simulink model "Test2"  (R2017b)
settings: Solver=ode23tb  StartTime=0.0  StopTime=6  MaxStep=1e-4  RelTol=1e-3
undefined symbols (not defined in the file): DiscIntNeverNeededParam
libraries: powerlib x5, simulink x1
settings Model: Creator=80573  LastModifiedBy=80573

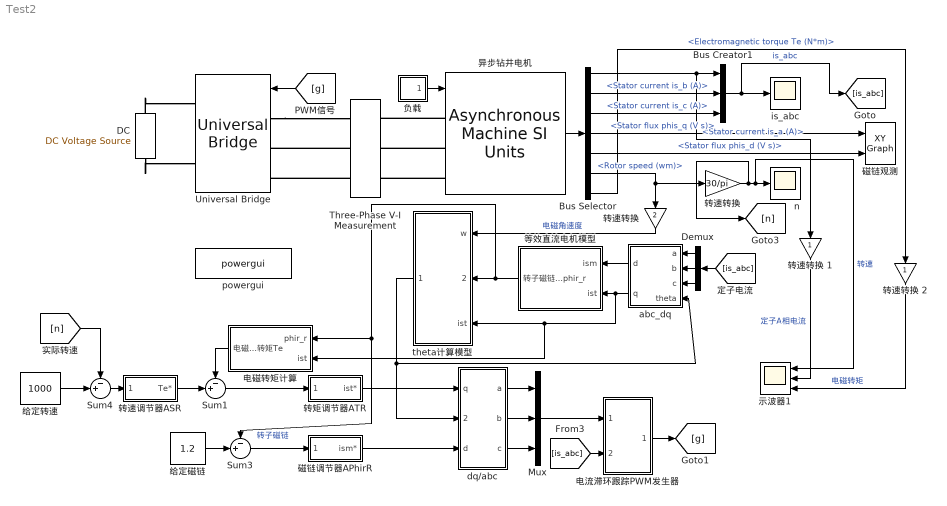
== system Test2 ==
  Bus Creator1 : BusCreator  Inputs=3
  Bus Selector : BusSelector  OutputSignals=Stator measurements.Stator current is_a (A),Stator measurements.Stator current is_b (A),Stator measurements.Stator current is_c (A),Stator measurements.Stator flux phis_q (V s),Stator measurements.Stator flux phis_d (V s),Mechanical.Rotor speed (wm),Mechanical.Electromagnetic torque Te (N*m)
  DC : powerlib/Electrical Sources/DC Voltage Source  Amplitude=510  Measurements=None
  Demux : Demux  Outputs=3
  Mux : Mux  Inputs=3
  Sum1 : Sum  Inputs=-+|
  Sum3 : Sum  Inputs=-+|
  Sum4 : Sum  Inputs=-+|
  Three-Phase V-I Measurement : powerlib/Measurements/Three-Phase V-I Measurement  VoltageMeasurement=phase-to-phase  SetLabelV=on  LabelV=Vabc  Vpu=off  VpuLL=off  CurrentMeasurement=yes  SetLabelI=on  LabelI=Iabc  Ipu=off  Pbase=100e6  Vbase=500e3  OutputType=Complex  PhasorSimulation=off  PSBequivalent=0
  Universal Bridge : powerlib/Power Electronics/Universal Bridge  Arms=3  SnubberResistance=1e5  SnubberCapacitance=inf  Device=IGBT / Diodes  Ron=1e-3  Lon=0  ForwardVoltages="[  0  0  ]"  ForwardVoltage=0  GTOparameters=[ 10e-6 , 20e-6 ]  IGBTparameters=[ 1e-6 , 2e-6 ]  Measurements=None  Measurements_2=None  converterType=Rectifier
  abc_dq : Subsystem
  dq/abc : Subsystem
  is_abc : Scope
  n : Scope
  powergui : powerlib/powergui  SimulationMode=Discrete  SampleTime=0.00001  frequency=50  Iterations=50  frequencyindice=0  Pbase=100e6  ErrMax=1e-4  UnitsV=kV  UnitsW=MW  buscounter=0  FunctionMessages=off  echomessages=off  EnableUseOfTLC=off  CurrentSourceSwitches=off  DisableSnubberDevices=off  DisableRonSwitches=off  DisableVfSwitches=off  DisplayEquations=off  SolverType=Tustin/Backward Euler (TBE)  Interpol=off  ExternalGateDelay=off  methode=off  Ts=100  x0status=zero  SPID=on  SwTol=0  HookPort=off  RestoreLinks=warning  ResistiveCurrentMeasurement=off  Frange=[0:2:500]  Ylog=off  Xlog=on  ShowGrid=off  save=off  variable=ZData  structure=0  ZoomFFT=on  StartTime=0.0  cycles=1  DisplayStyle=1  fundamental=60  FreqAxis=off  MaxFrequency=1000  frequencyindicesteady=1  RmsSteady=1  display=off
  theta计算模型 : Subsystem
  异步钻井电机 : powerlib/Machines/Asynchronous Machine SI Units  RotorType=Squirrel-cage  PresetModel=No  MechanicalLoad=Torque Tm  ShowDetailedParameters=on  ReferenceFrame=Stationary  Units=SI  MeasurementBus=off  NominalParameters=[149200 380 50]  Stator=[0.01485 0.0003027]  Rotor=[0.05295 0.0003027]  Cage1=[0.4155 0.002066]  Cage2=[0.4168 0.0003495]  Lm=0.01046  Mechanical=[3.1 0.08 2]  PolePairs=2  InitialConditions=[1 0 0 0 0 0 0 0]  SimulateSaturation=off  Saturation=[14.03593122, 27.81365428, 53.79336849, 72.68890987, 97.98006896, 148.6815601, 215.7428561, 302.9841135, 428.7778367 ; 230, 322, 414, 460, 506, 552, 598, 644, 690]  LoadFlowParameters=1492000  TsPowergui=0  TsBlock=-1  IterativeModel=Trapezoidal non iterative  IterativeDiscreteModel=Trapezoidal non iterative  Pmec=1.492e+006
  电流滞环跟踪PWM发生器 : Subsystem
  电磁转矩计算 : Subsystem
  磁链观测 : simulink/Sinks/XY Graph  xmin=-1  xmax=1  ymin=-1  ymax=1  st=-1
  磁链调节器APhirR : Subsystem
  示波器1 : Scope  NumInputPorts=3
  等效直流电机模型 : Subsystem
  给定磁链 : Constant  Value=1.2
  给定转速 : Constant  Value=1000
  负载 : Subsystem
  转矩调节器ATR : Subsystem
  转速调节器ASR : Subsystem
  转速转换 : Gain  Gain=30/pi
  "转速转换 " : Gain  Gain=2
  转速转换 1 : Gain
  转速转换 2 : Gain
  wires:
  Bus Selector/7 -> 转速转换 2/1  "<Electromagnetic torque Te (N*m)>"
  Demux/3 -> abc_dq/3(c)
  Sum1/1 -> 转矩调节器ATR/1(" ")
  转矩调节器ATR/1(ist*) -> dq/abc/1(q)
  [n] -> Sum4/1
  "转速转换 "/1 -> theta计算模型/1(w)  "电磁角速度"
  电流滞环跟踪PWM发生器/1(pulse) -> [g]
  Bus Selector/5 -> 磁链观测/2  "<Stator flux phis_d (V s)>"
  Sum4/1 -> 转速调节器ASR/1("  ")
  dq/abc/1(a) -> Mux/1
  转速转换/1 -> [n], 示波器1/1, n/1  "转速"
  dq/abc/2(b) -> Mux/2
  转速转换 2/1 -> 示波器1/3  "电磁转矩"
  异步钻井电机/1 -> Bus Selector/1
  theta计算模型/1(theta) -> dq/abc/2(theta), abc_dq/4(theta)
  Bus Selector/6 -> 转速转换/1, "转速转换 "/1  "<Rotor speed (wm)>"
  转速调节器ASR/1(Te*) -> Sum1/2
  Bus Selector/2 -> Bus Creator1/2  "<Stator current is_b (A)>"
  电磁转矩计算/1(电磁转矩Te) -> Sum1/1
  abc_dq/1(d) -> 等效直流电机模型/1(ism)
  负载/1(TL) -> 异步钻井电机/1
  Mux/1 -> 电流滞环跟踪PWM发生器/1(Iabc*)
  Demux/2 -> abc_dq/2(b)
  [is_abc] -> Demux/1
  [is_abc] -> 电流滞环跟踪PWM发生器/2(Iabc)
  dq/abc/3(c) -> Mux/3
  转速转换 1/1 -> 示波器1/2  "定子A相电流"
  Bus Selector/1 -> 转速转换 1/1, Bus Creator1/1  "<Stator current is_a (A)>"
  abc_dq/2(q) -> 等效直流电机模型/2(ist), theta计算模型/3(ist), 电磁转矩计算/2(ist)
  Bus Selector/3 -> Bus Creator1/3  "<Stator current is_c (A)>"
  Demux/1 -> abc_dq/1(a)
  给定磁链/1 -> Sum3/2
  Sum3/1 -> 磁链调节器APhirR/1(" ")
  Bus Selector/4 -> 磁链观测/1  "<Stator flux phis_q (V s)>"
  Bus Creator1/1 -> is_abc/1, [is_abc]  "is_abc"
  磁链调节器APhirR/1(ism*) -> dq/abc/3(d)
  [g] -> Universal Bridge/1
  等效直流电机模型/1(转子磁链phir_r) -> theta计算模型/2(phir_r), Sum3/1, 电磁转矩计算/1(phir_r)  "转子磁链"
  给定转速/1 -> Sum4/2
  connections:
  DC/LConn1 -- Universal Bridge/RConn2
  Three-Phase V-I Measurement/LConn3 -- Universal Bridge/LConn3
  异步钻井电机/LConn2 -- Three-Phase V-I Measurement/RConn2
  异步钻井电机/LConn3 -- Three-Phase V-I Measurement/RConn3
  Universal Bridge/LConn1 -- Three-Phase V-I Measurement/LConn1
  DC/RConn1 -- Universal Bridge/RConn1
  Three-Phase V-I Measurement/LConn2 -- Universal Bridge/LConn2
  异步钻井电机/LConn1 -- Three-Phase V-I Measurement/RConn1

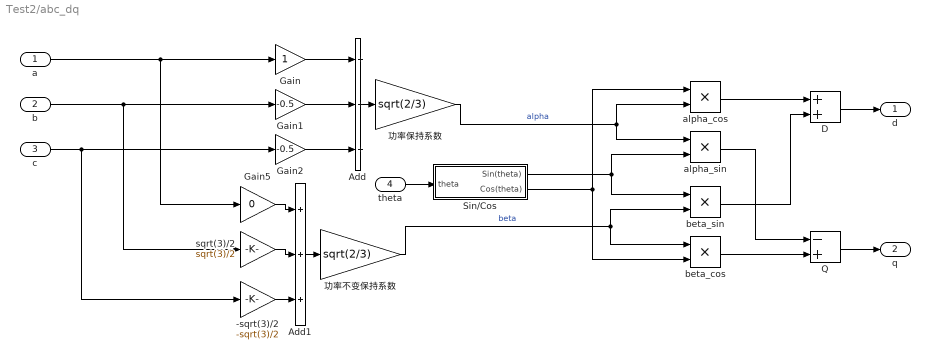
== system Test2/abc_dq ==
  a : Inport
  b : Inport  Port=2
  c : Inport  Port=3
  theta : Inport  Port=4
  -sqrt(3)/2 : Gain  Gain=-sqrt(3)/2
  Add : Sum  Inputs=3
  Add1 : Sum  Inputs=3
  D : Sum
  Gain : Gain
  Gain1 : Gain  Gain=-0.5
  Gain2 : Gain  Gain=-0.5
  Gain5 : Gain  Gain=0
  Q : Sum  Inputs=-+
  Sin/Cos : Subsystem
  alpha_cos : Product
  alpha_sin : Product
  beta_cos : Product
  beta_sin : Product
  sqrt(3)/2 : Gain  Gain=sqrt(3)/2
  功率不变保持系数 : Gain  Gain=sqrt(2/3)
  功率保持系数 : Gain  Gain=sqrt(2/3)
  d : Outport
  q : Outport  Port=2
  wires:
  功率不变保持系数/1 -> beta_cos/1, beta_sin/2  "beta"
  D/1 -> d/1
  Sin/Cos/2(Cos(theta)) -> beta_cos/2, alpha_cos/1
  alpha_sin/1 -> Q/1
  Q/1 -> q/1
  beta_sin/1 -> D/2
  beta_cos/1 -> Q/2
  Sin/Cos/1(Sin(theta)) -> beta_sin/1, alpha_sin/2
  功率保持系数/1 -> alpha_cos/2, alpha_sin/1  "alpha"
  Add1/1 -> 功率不变保持系数/1
  c/1 -> Gain2/1, -sqrt(3)/2/1
  a/1 -> Gain5/1, Gain/1
  Gain2/1 -> Add/3
  sqrt(3)/2/1 -> Add1/2
  theta/1 -> Sin/Cos/1(theta)
  b/1 -> sqrt(3)/2/1, Gain1/1
  -sqrt(3)/2/1 -> Add1/3
  Gain1/1 -> Add/2
  Gain5/1 -> Add1/1
  alpha_cos/1 -> D/1
  Add/1 -> 功率保持系数/1
  Gain/1 -> Add/1

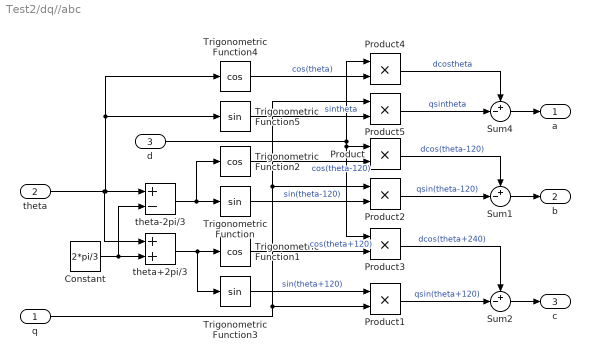
== system Test2/dq//abc ==
  q : Inport
  theta : Inport  Port=2
  d : Inport  Port=3
  Constant : Constant  Value=2*pi/3
  Product{,1..5} (6 alike) : Product
  Sum1 : Sum  Inputs=+-|
  Sum2 : Sum  Inputs=+-|
  Sum4 : Sum  Inputs=+-|
  Trigonometric Function : Trigonometry
  Trigonometric Function1 : Trigonometry  Operator=cos
  Trigonometric Function2 : Trigonometry  Operator=cos
  Trigonometric Function3 : Trigonometry
  Trigonometric Function4 : Trigonometry  Operator=cos
  Trigonometric Function5 : Trigonometry
  theta+2pi/3 : Sum
  theta-2pi/3 : Sum  Inputs=+-
  a : Outport
  b : Outport  Port=2
  c : Outport  Port=3
  wires:
  Trigonometric Function5/1 -> Product5/2  "sintheta"
  Product/1 -> Sum1/1  "dcos(theta-120)"
  Trigonometric Function1/1 -> Product3/2  "cos(theta+120)"
  Product3/1 -> Sum2/1  "dcos(theta+240)"
  d/1 -> Product/1, Product3/1, Product4/1
  Constant/1 -> theta+2pi/3/2, theta-2pi/3/2
  theta/1 -> Trigonometric Function4/1, Trigonometric Function5/1, theta-2pi/3/1, theta+2pi/3/1
  theta+2pi/3/1 -> Trigonometric Function3/1, Trigonometric Function1/1
  q/1 -> Product5/1, Product2/1, Product1/2
  Trigonometric Function/1 -> Product2/2  "sin(theta-120)"
  Product4/1 -> Sum4/1  "dcostheta"
  Product5/1 -> Sum4/2  "qsintheta"
  theta-2pi/3/1 -> Trigonometric Function2/1, Trigonometric Function/1
  Product1/1 -> Sum2/2  "qsin(theta+120)"
  Trigonometric Function2/1 -> Product/2  "cos(theta-120)"
  Sum4/1 -> a/1
  Sum1/1 -> b/1
  Trigonometric Function4/1 -> Product4/2  "cos(theta)"
  Trigonometric Function3/1 -> Product1/1  "sin(theta+120)"
  Product2/1 -> Sum1/2  "qsin(theta-120)"
  Sum2/1 -> c/1

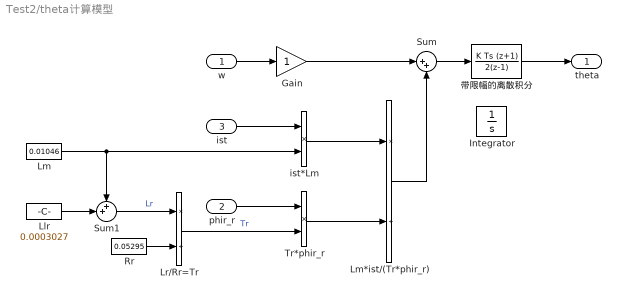
== system Test2/theta计算模型 ==
  w : Inport
  phir_r : Inport  Port=2
  ist : Inport  Port=3
  Gain : Gain
  Integrator : Integrator
  Llr : Constant  Value=0.0003027
  Lm : Constant  Value=0.01046
  Lm*ist/(Tr*phir_r) : Product  Inputs=*/
  Lr/Rr=Tr : Product  Inputs=*/
  Rr : Constant  Value=0.05295
  Sum : Sum  Inputs=|++
  Sum1 : Sum  Inputs=++|
  Tr*phir_r : Product
  ist*Lm : Product
  带限幅的离散积分 : DiscreteIntegrator  IntegratorMethod=Integration: Trapezoidal  SampleTime=2e-5  LimitOutput=on  UpperSaturationLimit=3000  LowerSaturationLimit=-3000  ICPrevOutput=DiscIntNeverNeededParam  ICPrevScaledInput=DiscIntNeverNeededParam
  theta : Outport
  wires:
  ist*Lm/1 -> Lm*ist/(Tr*phir_r)/1
  Lm*ist/(Tr*phir_r)/1 -> Sum/2
  Sum/1 -> 带限幅的离散积分/1
  w/1 -> Gain/1
  带限幅的离散积分/1 -> theta/1
  Lr/Rr=Tr/1 -> Tr*phir_r/2  "Tr"
  Lm/1 -> Sum1/1, ist*Lm/2
  Tr*phir_r/1 -> Lm*ist/(Tr*phir_r)/2
  ist/1 -> ist*Lm/1
  phir_r/1 -> Tr*phir_r/1
  Rr/1 -> Lr/Rr=Tr/2
  Gain/1 -> Sum/1
  Sum1/1 -> Lr/Rr=Tr/1  "Lr"
  Llr/1 -> Sum1/2

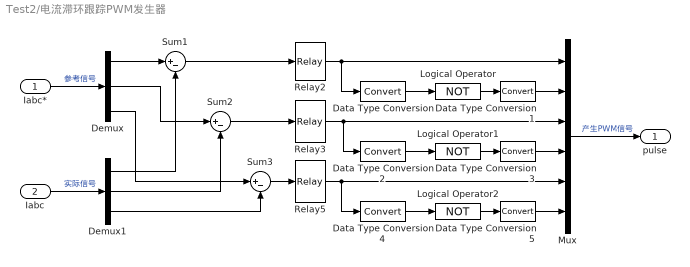
== system Test2/电流滞环跟踪PWM发生器 ==
  Iabc* : Inport
  Iabc : Inport  Port=2
  Data Type Conversion{,1..5} (6 alike) : DataTypeConversion
  Demux : Demux  Outputs=3
  Demux1 : Demux  Outputs=3
  Logical Operator : Logic  Operator=NOT  Inputs=1  AllPortsSameDT=off
  Logical Operator1 : Logic  Operator=NOT  Inputs=1  AllPortsSameDT=off
  Logical Operator2 : Logic  Operator=NOT  Inputs=1  AllPortsSameDT=off
  Mux : Mux  Inputs=6
  Relay2 : Relay  OnSwitchValue=0.2  OffSwitchValue=-0.2  ZeroCross=off
  Relay3 : Relay  OnSwitchValue=0.2  OffSwitchValue=-0.2  ZeroCross=off
  Relay5 : Relay  OnSwitchValue=0.2  OffSwitchValue=-0.2  ZeroCross=off
  Sum1 : Sum  Inputs=|+-
  Sum2 : Sum  Inputs=|+-
  Sum3 : Sum  Inputs=|+-
  pulse : Outport
  wires:
  Relay2/1 -> Data Type Conversion/1, Mux/1
  Data Type Conversion/1 -> Logical Operator/1
  Logical Operator/1 -> Data Type Conversion1/1
  Data Type Conversion1/1 -> Mux/2
  Mux/1 -> pulse/1  "产生PWM信号"
  Sum1/1 -> Relay2/1
  Demux/1 -> Sum1/1
  Demux1/3 -> Sum3/2
  Iabc/1 -> Demux1/1  "实际信号"
  Iabc*/1 -> Demux/1  "参考信号"
  Sum2/1 -> Relay3/1
  Logical Operator1/1 -> Data Type Conversion3/1
  Data Type Conversion3/1 -> Mux/4
  Data Type Conversion2/1 -> Logical Operator1/1
  Relay3/1 -> Data Type Conversion2/1, Mux/3
  Logical Operator2/1 -> Data Type Conversion5/1
  Data Type Conversion5/1 -> Mux/6
  Data Type Conversion4/1 -> Logical Operator2/1
  Relay5/1 -> Data Type Conversion4/1, Mux/5
  Sum3/1 -> Relay5/1
  Demux/2 -> Sum2/1
  Demux1/1 -> Sum1/2
  Demux1/2 -> Sum2/2
  Demux/3 -> Sum3/1

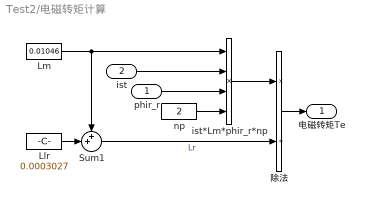
== system Test2/电磁转矩计算 ==
  phir_r : Inport
  ist : Inport  Port=2
  Llr : Constant  Value=0.0003027
  Lm : Constant  Value=0.01046
  Sum1 : Sum  Inputs=++|
  ist*Lm*phir_r*np : Product  Inputs=4
  np : Constant  Value=2
  除法 : Product  Inputs=*/
  电磁转矩Te : Outport
  wires:
  np/1 -> ist*Lm*phir_r*np/4
  phir_r/1 -> ist*Lm*phir_r*np/3
  除法/1 -> 电磁转矩Te/1
  ist*Lm*phir_r*np/1 -> 除法/1
  Sum1/1 -> 除法/2  "Lr"
  Llr/1 -> Sum1/2
  ist/1 -> ist*Lm*phir_r*np/2
  Lm/1 -> Sum1/1, ist*Lm*phir_r*np/1

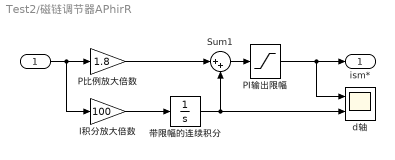
== system Test2/磁链调节器APhirR ==
  " " : Inport
  I积分放大倍数 : Gain  Gain=100
  PI输出限幅 : Saturate  UpperLimit=1300  LowerLimit=-1300
  P比例放大倍数 : Gain  Gain=1.8
  Sum1 : Sum  Inputs=|++
  d轴 : Scope  NumInputPorts=2
  带限幅的连续积分 : Integrator  LimitOutput=on  UpperSaturationLimit=1500  LowerSaturationLimit=-1500
  ism* : Outport
  wires:
  Sum1/1 -> PI输出限幅/1
  I积分放大倍数/1 -> 带限幅的连续积分/1
  P比例放大倍数/1 -> Sum1/1
  " "/1 -> I积分放大倍数/1, P比例放大倍数/1
  PI输出限幅/1 -> ism*/1, d轴/1
  带限幅的连续积分/1 -> d轴/2, Sum1/2

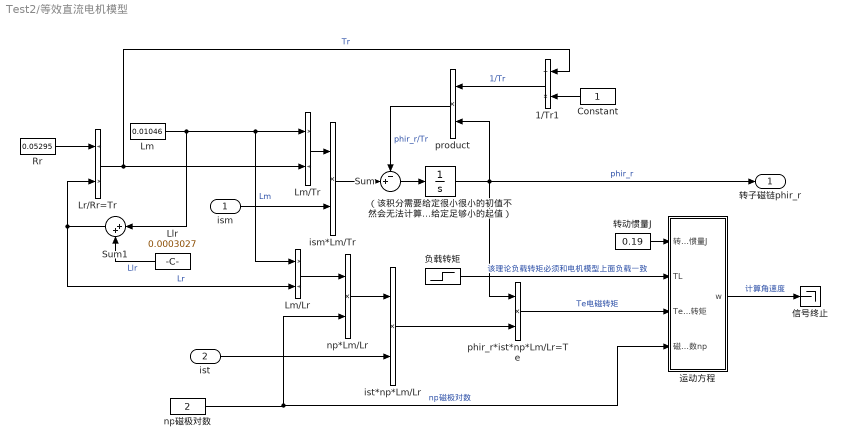
== system Test2/等效直流电机模型 ==
  ism : Inport
  ist : Inport  Port=2
  1/Tr1 : Product  Inputs=/*
  Constant : Constant
  Llr : Constant  Value=0.0003027
  Lm : Constant  Value=0.01046
  Lm/Lr : Product  Inputs=*/
  Lm/Tr : Product  Inputs=*/
  Lr/Rr=Tr : Product  Inputs=/*
  Rr : Constant  Value=0.05295
  Sum : Sum  Inputs=-+|
  Sum1 : Sum  Inputs=|++
  ism*Lm/Tr : Product
  ist*np*Lm/Lr : Product
  np*Lm/Lr : Product
  np磁极对数 : Constant  Value=2
  phir_r*ist*np*Lm/Lr=Te : Product
  product : Product
  信号终止 : Terminator
  负载转矩 : Step  Time=0.6  After=55  SampleTime=0
  转动惯量J : Constant  Value=0.19
  运动方程 : Subsystem
  （该积分需要给定很小很小的初值不然会无法计算 原因是数学推导中积分起值为0所以一直都为0 所以要能够计算必须给定足够小的起值） : Integrator  InitialCondition=1e-5
  转子磁链phir_r : Outport
  wires:
  ism/1 -> ism*Lm/Tr/2
  Sum/1 -> （该积分需要给定很小很小的初值不然会无法计算 原因是数学推导中积分起值为0所以一直都为0 所以要能够计算必须给定足够小的起值）/1
  转动惯量J/1 -> 运动方程/1(转动惯量J)
  运动方程/1(w) -> 信号终止/1  "计算角速度"
  phir_r*ist*np*Lm/Lr=Te/1 -> 运动方程/3(Te电磁转矩)  "Te电磁转矩"
  负载转矩/1 -> 运动方程/2(TL)  "该理论负载转矩必须和电机模型上面负载一致"
  np*Lm/Lr/1 -> ist*np*Lm/Lr/1
  Lm/1 -> Sum1/1, Lm/Lr/1, Lm/Tr/1  "Lm"
  Lm/Tr/1 -> ism*Lm/Tr/1
  ist*np*Lm/Lr/1 -> phir_r*ist*np*Lm/Lr=Te/2
  ism*Lm/Tr/1 -> Sum/2
  product/1 -> Sum/1  "phir_r/Tr"
  ist/1 -> ist*np*Lm/Lr/2
  np磁极对数/1 -> np*Lm/Lr/2, 运动方程/4(磁极对数np)  "np磁极对数"
  Lm/Lr/1 -> np*Lm/Lr/1
  （该积分需要给定很小很小的初值不然会无法计算 原因是数学推导中积分起值为0所以一直都为0 所以要能够计算必须给定足够小的起值）/1 -> 转子磁链phir_r/1, product/2, phir_r*ist*np*Lm/Lr=Te/1  "phir_r"
  1/Tr1/1 -> product/1  "1/Tr"
  Lr/Rr=Tr/1 -> Lm/Tr/2, 1/Tr1/1  "Tr"
  Rr/1 -> Lr/Rr=Tr/1
  Constant/1 -> 1/Tr1/2
  Sum1/1 -> Lm/Lr/2, Lr/Rr=Tr/2  "Lr"
  Llr/1 -> Sum1/2  "Llr"

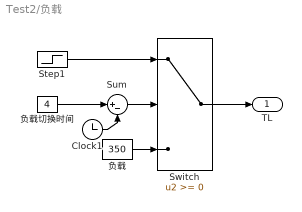
== system Test2/负载 ==
  Clock1 : Clock
  Step1 : Step  Time=2  Before=200  After=500  SampleTime=0
  Sum : Sum  Inputs=|+-
  Switch : Switch
  负载 : Constant  Value=350
  负载切换时间 : Constant  Value=4
  TL : Outport
  wires:
  Clock1/1 -> Sum/2
  Switch/1 -> TL/1
  Sum/1 -> Switch/2
  负载/1 -> Switch/3
  负载切换时间/1 -> Sum/1
  Step1/1 -> Switch/1

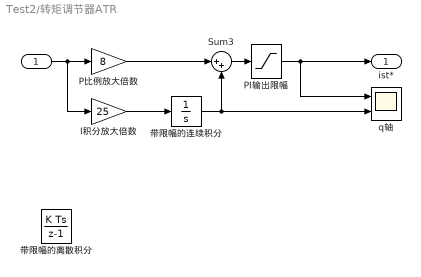
== system Test2/转矩调节器ATR ==
  " " : Inport
  I积分放大倍数 : Gain  Gain=25
  PI输出限幅 : Saturate  UpperLimit=500  LowerLimit=-500
  P比例放大倍数 : Gain  Gain=8
  Sum3 : Sum  Inputs=|++
  "q轴 " : Scope  NumInputPorts=2
  带限幅的离散积分 : DiscreteIntegrator  SampleTime=2e-5  ICPrevOutput=DiscIntNeverNeededParam  ICPrevScaledInput=DiscIntNeverNeededParam
  带限幅的连续积分 : Integrator  LimitOutput=on  UpperSaturationLimit=510  LowerSaturationLimit=-510
  ist* : Outport
  wires:
  Sum3/1 -> PI输出限幅/1
  P比例放大倍数/1 -> Sum3/1
  " "/1 -> I积分放大倍数/1, P比例放大倍数/1
  I积分放大倍数/1 -> 带限幅的连续积分/1
  PI输出限幅/1 -> ist*/1, "q轴 "/1
  带限幅的连续积分/1 -> "q轴 "/2, Sum3/2

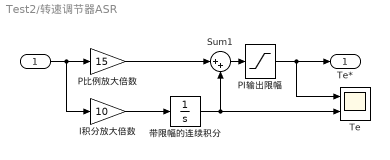
== system Test2/转速调节器ASR ==
  "  " : Inport
  I积分放大倍数 : Gain  Gain=10
  PI输出限幅 : Saturate  UpperLimit=500  LowerLimit=-500
  P比例放大倍数 : Gain  Gain=15
  Sum1 : Sum  Inputs=|++
  Te : Scope  NumInputPorts=2
  带限幅的连续积分 : Integrator  LimitOutput=on  UpperSaturationLimit=510  LowerSaturationLimit=-510
  Te* : Outport
  wires:
  Sum1/1 -> PI输出限幅/1
  PI输出限幅/1 -> Te*/1, Te/1
  P比例放大倍数/1 -> Sum1/1
  I积分放大倍数/1 -> 带限幅的连续积分/1
  带限幅的连续积分/1 -> Te/2, Sum1/2
  "  "/1 -> I积分放大倍数/1, P比例放大倍数/1

== system Test2/abc_dq/Sin//Cos ==
  theta : Inport
  cos : Trigonometry  Operator=cos
  sin : Trigonometry
  Sin(theta) : Outport
  Cos(theta) : Outport  Port=2
  wires:
  sin/1 -> Sin(theta)/1
  theta/1 -> sin/1, cos/1
  cos/1 -> Cos(theta)/1

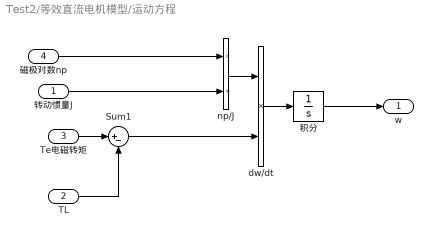
== system Test2/等效直流电机模型/运动方程 ==
  转动惯量J : Inport
  TL : Inport  Port=2
  Te电磁转矩 : Inport  Port=3
  磁极对数np : Inport  Port=4
  Sum1 : Sum  Inputs=|+-
  dw/dt : Product
  np/J : Product  Inputs=*/
  积分 : Integrator
  w : Outport
  wires:
  转动惯量J/1 -> np/J/2
  Sum1/1 -> dw/dt/2
  TL/1 -> Sum1/2
  积分/1 -> w/1
  磁极对数np/1 -> np/J/1
  np/J/1 -> dw/dt/1
  Te电磁转矩/1 -> Sum1/1
  dw/dt/1 -> 积分/1
